simulink model "hybrid_version"  (R2022a)
settings: Solver=VariableStepAuto  StartTime=0.0  StopTime=2  MaxStep=0.01  RelTol=1e-3
values from neighbouring files (symbols this model uses):
  k_gn = m*g/0.001    (= 412020)    [controller_parameters.m]
  k_gt = m*g/0.1    (= 4120.2)    [controller_parameters.m]
  m = 42    [controller_parameters.m]    (also in ground_reaction_params.m = 12)
  mu_slide = 0.8    [controller_parameters.m]    (also in ground_reaction_params.m = 0.008)
  mu_stick = 0.9    [controller_parameters.m]    (also in ground_reaction_params.m = 0.009)
  v_gn_max = 0.03    [controller_parameters.m]
  v_gt_max = 0.03    [controller_parameters.m]
  vLimit = 0.01    [controller_parameters.m]    (also in ground_reaction_params.m = 0.001)
undefined symbols (not defined in the file or in its folder): Newton, Raphson, X, Y, Z
libraries: sm_lib x179, nesl_utility x110, simulink x32, simulink_extras x8
(part 1 of 8)
settings Model: Creator=nemo  LastModifiedBy=prass

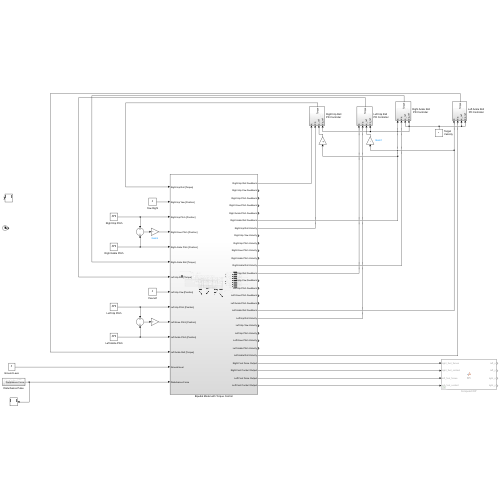
[thumbnail: Simulink's stored preview of the top-level diagram]
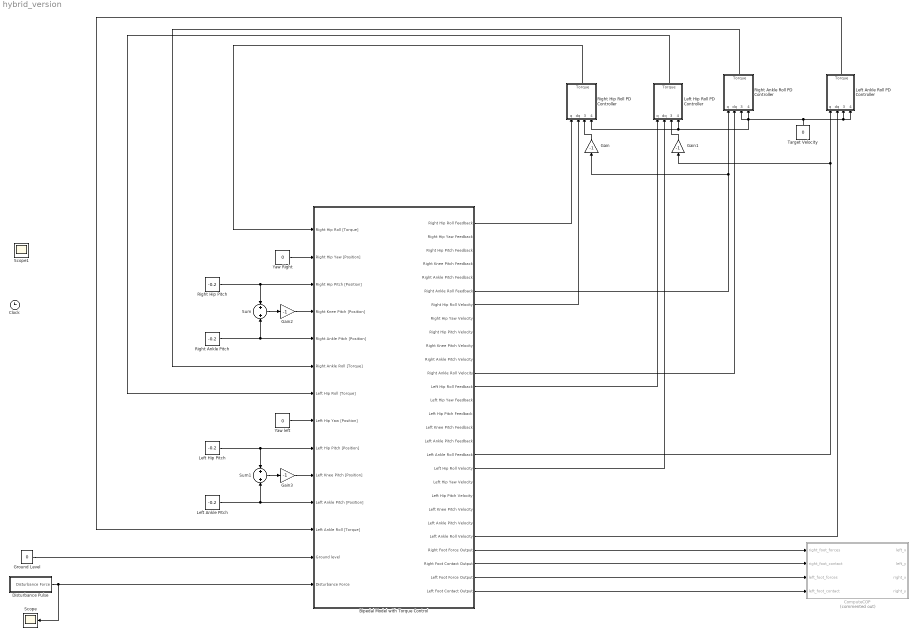
== system hybrid_version ==
  " Left Ankle Pitch" : Constant  Value=-0.2
  " Left Hip Pitch" : Constant  Value=-0.2
  " Right Ankle Pitch" : Constant  Value=-0.2
  " Right Hip Pitch" : Constant  Value=-0.2
  Bipedal Model with Torque Control : Subsystem
  Clock : Clock
  "ComputeCOP " : MATLAB Function  Commented=on  TreatAsAtomicUnit=on
  Disturbance Pulse : Subsystem
  Gain{,1..3} (4 alike) : Gain  Gain=-1
  Ground Level : Constant  Value=0
  Left Ankle Roll PD Controller : Subsystem
  Left Hip Roll PD Controller : Subsystem
  Right Ankle Roll PD Controller : Subsystem
  Right Hip Roll PD Controller : Subsystem
  Scope : Scope
  Scope1 : Scope
  Sum : Sum
  Sum1 : Sum
  Target Velocity : Constant  Value=0
  Yaw Right : Constant  Value=0
  Yaw left : Constant  Value=0
  wires:
  Disturbance Pulse/1(Disturbance Force) -> Bipedal Model with Torque Control/14(Disturbance Force), Scope/1
  Ground Level/1 -> Bipedal Model with Torque Control/13(Ground level)
  Bipedal Model with Torque Control/25(Right Foot Force Output) -> "ComputeCOP "/1(right_foot_forces)
  Bipedal Model with Torque Control/26(Right Foot Contact Output) -> "ComputeCOP "/2(right_foot_contact)
  Bipedal Model with Torque Control/28(Left Foot Contact Output) -> "ComputeCOP "/4(left_foot_contact)
  Bipedal Model with Torque Control/27(Left Foot Force Output) -> "ComputeCOP "/3(left_foot_forces)
  Bipedal Model with Torque Control/6(Right Ankle Roll Feedback) -> Gain/1, Right Ankle Roll PD Controller/1(q)
  Bipedal Model with Torque Control/12(Right Ankle Roll Velocity) -> Right Ankle Roll PD Controller/2(dq)
  Right Ankle Roll PD Controller/1(Torque) -> Bipedal Model with Torque Control/6(Right Ankle Roll [Torque])
  Bipedal Model with Torque Control/18(Left Ankle Roll Feedback) -> Gain1/1, Left Ankle Roll PD Controller/1(q)
  Left Ankle Roll PD Controller/1(Torque) -> Bipedal Model with Torque Control/12(Left Ankle Roll [Torque])
  Bipedal Model with Torque Control/24(Left Ankle Roll Velocity) -> Left Ankle Roll PD Controller/2(dq)
  Target Velocity/1 -> Right Hip Roll PD Controller/4(dq_ref), Left Hip Roll PD Controller/4(dq_ref), Right Ankle Roll PD Controller/3(q_ref), Right Ankle Roll PD Controller/4(dq_ref), Left Ankle Roll PD Controller/4(dq_ref), Left Ankle Roll PD Controller/3(q_ref)
  Right Hip Roll PD Controller/1(Torque) -> Bipedal Model with Torque Control/1(Right Hip Roll [Torque])
  Left Hip Roll PD Controller/1(Torque) -> Bipedal Model with Torque Control/7(Left Hip Roll [Torque])
  Bipedal Model with Torque Control/1(Right Hip Roll Feedback) -> Right Hip Roll PD Controller/1(q)
  Bipedal Model with Torque Control/7(Right Hip Roll Velocity) -> Right Hip Roll PD Controller/2(dq)
  Bipedal Model with Torque Control/13(Left Hip Roll Feedback) -> Left Hip Roll PD Controller/1(q)
  Bipedal Model with Torque Control/19(Left Hip Roll Velocity) -> Left Hip Roll PD Controller/2(dq)
  Gain1/1 -> Left Hip Roll PD Controller/3(q_ref)
  Gain/1 -> Right Hip Roll PD Controller/3(q_ref)
  Yaw Right/1 -> Bipedal Model with Torque Control/2(Right Hip Yaw [Position])
  Yaw left/1 -> Bipedal Model with Torque Control/8(Left Hip Yaw [Position])
  Sum/1 -> Gain2/1
  Gain2/1 -> Bipedal Model with Torque Control/4(Right Knee Pitch [Position])
  " Right Hip Pitch"/1 -> Sum/1, Bipedal Model with Torque Control/3(Right Hip Pitch [Position])
  " Right Ankle Pitch"/1 -> Sum/2, Bipedal Model with Torque Control/5(Right Ankle Pitch [Position])
  Sum1/1 -> Gain3/1
  " Left Hip Pitch"/1 -> Bipedal Model with Torque Control/9(Left Hip Pitch [Position]), Sum1/1
  " Left Ankle Pitch"/1 -> Bipedal Model with Torque Control/11(Left Ankle Pitch [Position]), Sum1/2
  Gain3/1 -> Bipedal Model with Torque Control/10(Left Knee Pitch [Position])
